simulink model "Lab_5_Real_System"  (R2019b)
settings: Solver=ode45  StartTime=0.0  StopTime=240  MaxStep=0.001  RelTol=1e-6  AbsTol=1e-4
values from neighbouring files (symbols this model uses):
  alpha = 0    [procedure_5_1.m]    (also in procedure_5_2.m; procedure_5_3.m)
  delay = 6    [shared_variables.m]
  desired_offset = -5    [shared_variables.m]
  frequency = 100    [shared_variables.m]
  K = 0    [procedure_5_1.m]
  T = 0    [procedure_5_1.m]    (also in procedure_5_2.m; procedure_5_3.m)
libraries: dspsigops x2
settings Model: DataDictionary=Lab_5_Real_System_Data.sldd  Creator=rolle  LastModifiedBy=rollends
settings SolverCC: ShapePreserveControl=EnableAll  ZeroCrossAlgorithm=Adaptive
settings DataIOCC: SaveOutput=off  DSMLogging=off  SaveTime=off  ReturnWorkspaceOutputs=off
settings DebuggingCC: IgnoredZcDiagnostic=none

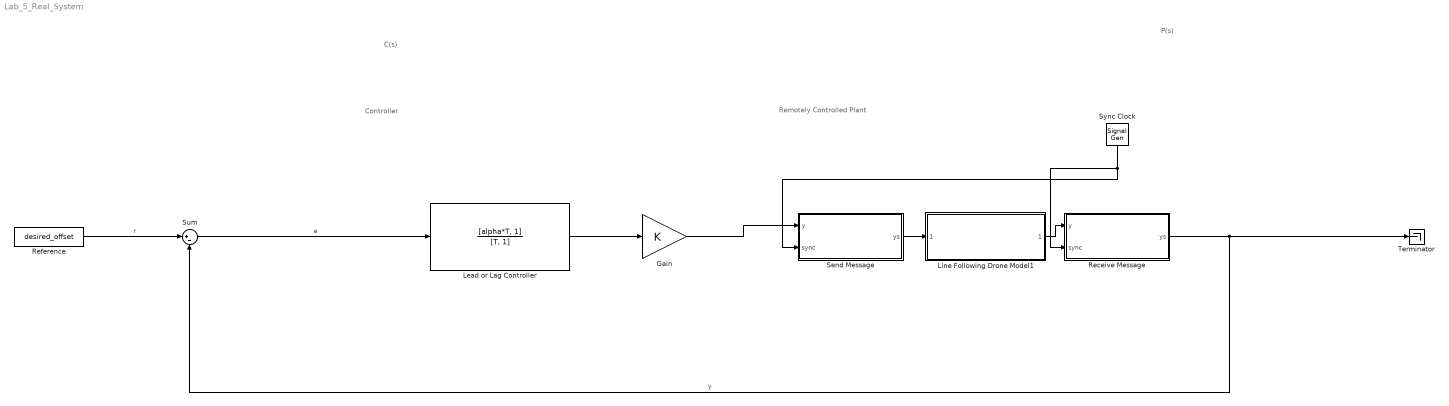
== system Lab_5_Real_System ==
  note: Controller
  note: P(s)
  note: Remotely Controlled Plant
  note: C(s)
  Gain : Gain  Gain=K
  Lead or Lag Controller : TransferFcn  Numerator=[alpha*T, 1]  Denominator=[T, 1]
  Line Following Drone Model1 : Subsystem  ReferencedSubsystem=Line_Following_Drone_Model
  Receive Message : Subsystem
  Reference : Constant  Value=desired_offset  OutDataTypeStr=Inherit: Inherit via back propagation
  Send Message : Subsystem
  Sum : Sum  Inputs=|+-
  Sync Clock : SignalGenerator  WaveForm=square  Frequency=frequency
  Terminator : Terminator
  wires:
  Reference/1 -> Sum/1  "r"
  Sum/1 -> Lead or Lag Controller/1  "e"
  Sync Clock/1 -> Send Message/2(sync), Receive Message/2(sync)
  Receive Message/1(ys) -> Sum/2, Terminator/1  "y"
  Lead or Lag Controller/1 -> Gain/1
  Gain/1 -> Send Message/1(y)
  Line Following Drone Model1/1 -> Receive Message/1(y)
  Send Message/1(ys) -> Line Following Drone Model1/1

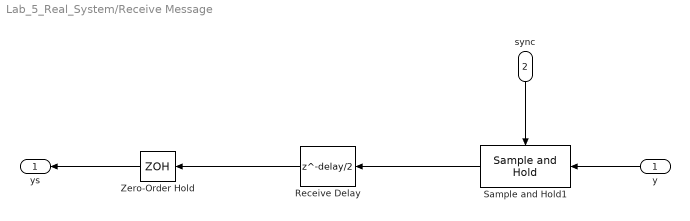
== system Lab_5_Real_System/Receive Message ==
  y : Inport
  sync : Inport  Port=2
  Receive Delay : Delay  DelayLength=delay/2  InitialCondition=0
  Sample and Hold1 : dspsigops/Sample and Hold  trig=Rising edge  initCond=0  latchinput=on
  Zero-Order Hold : ZeroOrderHold  SampleTime=-1
  ys : Outport
  wires:
  Receive Delay/1 -> Zero-Order Hold/1
  Zero-Order Hold/1 -> ys/1
  Sample and Hold1/1 -> Receive Delay/1
  y/1 -> Sample and Hold1/1
  sync/1 -> Sample and Hold1/Trigger

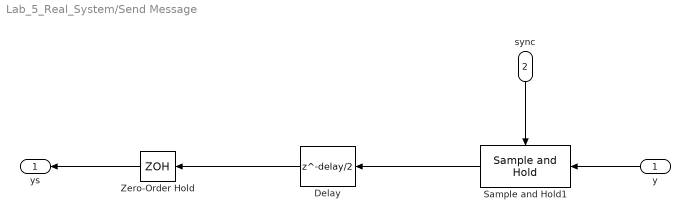
== system Lab_5_Real_System/Send Message ==
  y : Inport
  sync : Inport  Port=2
  Delay : Delay  DelayLength=delay/2  InitialCondition=0
  Sample and Hold1 : dspsigops/Sample and Hold  trig=Rising edge  initCond=0  latchinput=on
  Zero-Order Hold : ZeroOrderHold  SampleTime=-1
  ys : Outport
  wires:
  Delay/1 -> Zero-Order Hold/1
  Zero-Order Hold/1 -> ys/1
  Sample and Hold1/1 -> Delay/1
  y/1 -> Sample and Hold1/1
  sync/1 -> Sample and Hold1/Trigger
